simulink model "PVmodule"  (R2021a)
settings: Solver=VariableStepAuto  StartTime=0.0  StopTime=2.5  RelTol=1e-3
libraries: spsSeriesRLCBranchLib x2, pid_lib x2, spsMeanLib x2, spsDCVoltageSourceLib x1, spsDiodeLib x1, spsIGBTLib x1, eePwmGenerator x1, spsPVArrayLib x1, spsVoltageMeasurementLib x1, spspowerguiLib x1, SignalEditorBlockLib x1
settings Model: Creator=XieWHirlwind_TB  LastModifiedBy=XieWHirlwind_TB

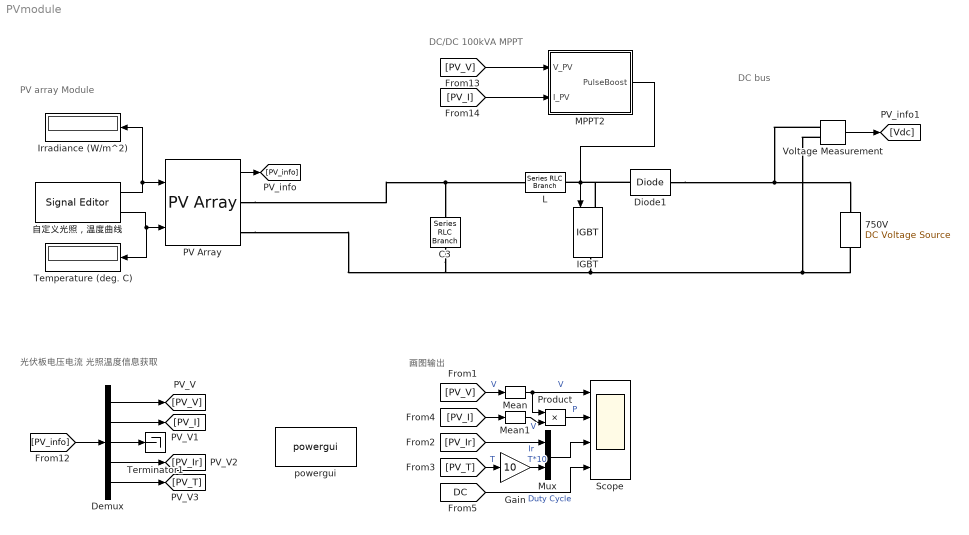
== system PVmodule ==
  note: DC bus
  note: 画图输出
  note: DC/DC 100kVA MPPT
  note: PV array Module
  note: 光伏板电压电流
      | 光照温度信息获取
  750V : spsDCVoltageSourceLib/DC Voltage Source  Amplitude=750  Measurements=None
  C3 : spsSeriesRLCBranchLib/Series RLC Branch  LConnTagsString=__new0  RConnTagsString=__new0  BranchType=C  Resistance=1.0  Inductance=1.0  SetiL0=off  InitialCurrent=0  Capacitance=470e-6  Setx0=off  InitialVoltage=0  Measurements=Branch voltage
  Demux : Demux  Outputs=5
  Diode1 : spsDiodeLib/Diode  Ron=1e-3  Lon=0  Vf=0.7  IC=0  UseSnubber=off  Rs=inf  Cs=inf  Measurements=off
  Gain : Gain  Gain=10
  IGBT : spsIGBTLib/IGBT  Ron=1e-3  Lon=0  Vf=0.7  Tf=1e-6  Tt=2e-6  IC=0  Rs=1e5  Cs=inf  Measurements=off
  Irradiance (W/m^2) : Display
      settings: Format=bank  Decimation=1000
  L : spsSeriesRLCBranchLib/Series RLC Branch  LConnTagsString=__new0  RConnTagsString=__new0  BranchType=RL  Resistance=0.0005  Inductance=1e-3  SetiL0=off  InitialCurrent=0  Capacitance=1e-6  Setx0=off  InitialVoltage=0  Measurements=None
  MPPT2 : Subsystem
  Mean : spsMeanLib/Mean  Freq=1e3  Vinit=0  Ts=1e-4
  Mean1 : spsMeanLib/Mean  Freq=1e3  Vinit=0  Ts=1e-4
  Mux : Mux  Inputs=2
  PV Array : spsPVArrayLib/PV Array  Npar=45  Nser=10  PlotType=array @ 25 deg.C & specified irradiances  S_vec="[ 1000 800 350  100 ]"  Temp_C_vec="[ 45 25  ]"  ModuleName=A2Peak Power POWER ON P220-6x10  PlotWhenSelected=off  Pm=219.978  Ncell=60  Voc=36.72  Isc=7.98  Vm=30.3  Im=7.26  beta_Voc_pc=-0.35  alpha_Isc_pc=0.05  beta_Voc=-0.12852  alpha_Isc=0.00399  IL=8.0041  I0=1.8441e-10  nI=0.97472  Rsh=85.0716  Rs=0.25728  RobustModel=off  RobustCellTemperature=313.3991  BAL=on  Tc=1e-6  Tfilter=5e-5
  Product : Product
  Scope : Scope  NumInputPorts=4
  Temperature (deg. C) : Display
      settings: Format=bank  Decimation=1000
  Terminator1 : Terminator
  Voltage Measurement : spsVoltageMeasurementLib/Voltage Measurement  PhasorSimulation=off  OutputType=Complex  PSBequivalent=0
  powergui : spspowerguiLib/powergui  Priority=1  SimulationMode=Discrete  SampleTime=2e-6  frequency=60  Iterations=50  frequencyindice=0  Pbase=100e6  ErrMax=1e-4  UnitsV=kV  UnitsW=MW  buscounter=0  FunctionMessages=off  echomessages=off  EnableUseOfTLC=off  CurrentSourceSwitches=off  DisableSnubberDevices=off  DisableRonSwitches=off  DisableVfSwitches=off  DisplayEquations=off  AutomaticDiscreteSolvers=off  SolverType=Tustin/Backward Euler (TBE)  Interpol=off  ExternalGateDelay=off  methode=off  Ts=100  x0status=blocks  SPID=on  SwTol=0  HookPort=off  NonlinearTolerance=1e-4  nMaxIteration=100  ContinueOnMaxIteration=off  RestoreLinks=warning  ResistiveCurrentMeasurement=off  Frange=[0:2:500]  Ylog=off  Xlog=on  ShowGrid=off  save=off  variable=ZData  structure=0  ZoomFFT=off  StartTime=0.0  cycles=1  DisplayStyle=1  fundamental=60  FreqAxis=off  MaxFrequency=1000  frequencyindicesteady=1  RmsSteady=1  display=off
  自定义光照，温度曲线 : SignalEditorBlockLib/Signal Editor  FileName=Irr_Temp_1.mat  ActiveScenario=Scenario1  ActiveSignal=Temp  IsBus=off  OutputBusObjectStr=Bus: BusObject  SampleTime=0  ZeroCross=off  OutputAfterFinalValue=Setting to zero  Unit=inherit  PreserveSignalName=on
  wires:
  MPPT2/1(PulseBoost) -> IGBT/1
  [PV_V] -> MPPT2/1(V_PV)
  自定义光照，温度曲线/2 -> Temperature (deg. C)/1, PV Array/2
  PV Array/1 -> [PV_info]
  自定义光照，温度曲线/1 -> Irradiance (W/m^2)/1, PV Array/1
  Demux/3 -> Terminator1/1
  Demux/4 -> [PV_Ir]
  Demux/5 -> [PV_T]
  [PV_info] -> Demux/1
  Demux/1 -> [PV_V]
  Demux/2 -> [PV_I]
  [PV_Ir] -> Mux/1  "Ir"
  Voltage Measurement/1 -> [Vdc]
  [PV_I] -> MPPT2/2(I_PV)
  Mean/1 -> Product/1, Scope/1  "V"
  [PV_V] -> Mean/1  "V"
  [PV_I] -> Mean1/1
  Product/1 -> Scope/2  "P"
  Mean1/1 -> Product/2  "V"
  Mux/1 -> Scope/3
  [DC] -> Scope/4  "Duty Cycle"
  [PV_T] -> Gain/1  "T"
  Gain/1 -> Mux/2  "T*10"
  connections:
  IGBT/RConn1 -- C3/RConn1 -- PV Array/RConn2 -- Voltage Measurement/LConn2 -- 750V/LConn1
  L/RConn1 -- IGBT/LConn1 -- Diode1/LConn1
  Diode1/RConn1 -- Voltage Measurement/LConn1 -- 750V/RConn1
  PV Array/RConn1 -- L/LConn1 -- C3/LConn1

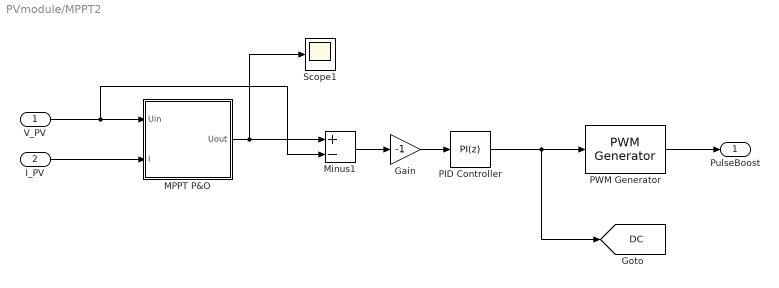
== system PVmodule/MPPT2 ==
  V_PV : Inport
  I_PV : Inport  Port=2
  Gain : Gain  Gain=-1
  MPPT P&O : Subsystem
  Minus1 : Sum  Inputs=+-
  PID Controller : pid_lib/PID Controller  Controller=PI  Form=Parallel  TimeDomain=Discrete-time  UseExternalTs=off  SampleTime=1e-4  IntegratorMethod=Forward Euler  FilterMethod=Forward Euler  ControllerParametersSource=internal  P=0.001  I=0.1  D=0  UseFilter=on  N=100  TunerSelectOption=Transfer Function Based (PID Tuner App)  InitialConditionSource=internal  InitialConditionForIntegrator=0  InitialConditionForFilter=0  DifferentiatorICPrevScaledInput=0  ExternalReset=none  TrackingMode=off  Kt=1  LimitOutput=on  SatLimitsSource=internal  UpperSaturationLimit=1  LowerSaturationLimit=0  LinearizeAsGain=on  AntiWindupMode=none  Kb=1  POutMin=[]  POutMax=[]  IOutMin=[]  IOutMax=[]  DOutMin=[]  DOutMax=[]  NOutMin=[]  NOutMax=[]  SumOutMin=[]  SumOutMax=[]  SaturationOutMin=[]  SaturationOutMax=[]  PParamMin=[]  PParamMax=[]  IParamMin=[]  IParamMax=[]  DParamMin=[]  DParamMax=[]  NParamMin=[]  NParamMax=[]  KbParamMin=[]  KbParamMax=[]  KtParamMin=[]  KtParamMax=[]  KbOutMin=[]  KbOutMax=[]  KtOutMin=[]  KtOutMax=[]  IntegratorOutMin=[]  IntegratorOutMax=[]  FilterOutMin=[]  FilterOutMax=[]  SumI1OutMin=[]  SumI1OutMax=[]  SumI2OutMin=[]  SumI2OutMax=[]  SumI3OutMin=[]  SumI3OutMax=[]  SumI4OutMin=[]  SumI4OutMax=[]  SumDOutMin=[]  SumDOutMax=[]  DifferentiatorOutMin=[]  DifferentiatorOutMax=[]  FilterDiffOutCoefMin=[]  FilterDiffOutCoefMax=[]  ReciprocalOutMin=[]  ReciprocalOutMax=[]  SumDenOutMin=[]  SumDenOutMax=[]  SumNumOutMin=[]  SumNumOutMax=[]  DivideOutMin=[]  DivideOutMax=[]  UdiffTsProdOutMin=[]  UdiffTsProdOutMax=[]  NTsProdOutMin=[]  NTsProdOutMax=[]  UintegralTsProdOutMin=[]  UintegralTsProdOutMax=[]  UngainTsProdOutMin=[]  UngainTsProdOutMax=[]  IntegratorContinuousStateAttributes=''  IntegratorStateMustResolveToSignalObject=off  IntegratorRTWStateStorageClass=Auto  FilterContinuousStateAttributes=''  FilterStateMustResolveToSignalObject=off  FilterRTWStateStorageClass=Auto  ParallelPVariant=InternalParameters  IdealPVariant=Disabled  IVariant=InternalParameters  DVariant=Disabled  IntegratorVariant=Discrete  SatVariant=Enabled  AWVariant=Passthrough  PCopyVariant=Disabled  TRVariant=Disabled  FdbkBlocksVariant=Forward  IdealPFdbkVariant=Disabled  SatFdbkVariant=Disabled  DerivativeFilterVariant=Disabled  NVariant=Disabled  NCopyVariant=Disabled_SignalSpec  FilterICVariant=Disabled  IntegratorICVariant=InternalICs  ExternalResetVariant=Disabled  TRSumVariant=Passthrough  SumFdbkVariant=Disabled  SumVariant=Sum_PI  TsampFilterVariant=InternalTs  TsampNgainVariant=Passthrough  TsampIntegralVariant=Passthrough  ExternalSaturationOutDataTypeStr=Inherit: Same as second input
  PWM Generator : eePwmGenerator/PWM Generator  CarrCount=Up  Tper=1e-4  Ts=2e-6
  Scope1 : Scope
  PulseBoost : Outport
  tag scope: DC=global
  wires:
  PWM Generator/1 -> PulseBoost/1
  I_PV/1 -> MPPT P&O/2(I)
  V_PV/1 -> Minus1/2, MPPT P&O/1(Uin)
  MPPT P&O/1(Uout) -> Minus1/1, Scope1/1
  Minus1/1 -> Gain/1
  PID Controller/1 -> [DC], PWM Generator/1
  Gain/1 -> PID Controller/1

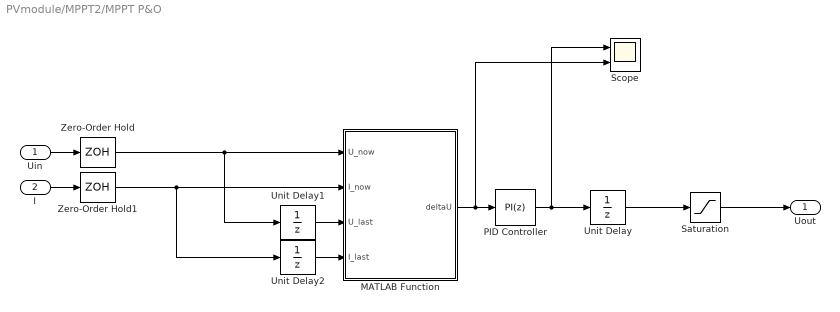
== system PVmodule/MPPT2/MPPT P&O ==
  Uin : Inport
  I : Inport  Port=2
  MATLAB Function : MATLAB Function  TreatAsAtomicUnit=on
  PID Controller : pid_lib/PID Controller  Controller=PI  Form=Parallel  TimeDomain=Discrete-time  UseExternalTs=off  SampleTime=1e-3  IntegratorMethod=Forward Euler  FilterMethod=Forward Euler  ControllerParametersSource=internal  P=1  I=100  D=0  UseFilter=on  N=100  TunerSelectOption=Transfer Function Based (PID Tuner App)  InitialConditionSource=internal  InitialConditionForIntegrator=250  InitialConditionForFilter=0  DifferentiatorICPrevScaledInput=0  ExternalReset=none  TrackingMode=off  Kt=1  LimitOutput=off  SatLimitsSource=internal  UpperSaturationLimit=inf  LowerSaturationLimit=-inf  LinearizeAsGain=on  AntiWindupMode=none  Kb=1  POutMin=[]  POutMax=[]  IOutMin=[]  IOutMax=[]  DOutMin=[]  DOutMax=[]  NOutMin=[]  NOutMax=[]  SumOutMin=[]  SumOutMax=[]  SaturationOutMin=[]  SaturationOutMax=[]  PParamMin=[]  PParamMax=[]  IParamMin=[]  IParamMax=[]  DParamMin=[]  DParamMax=[]  NParamMin=[]  NParamMax=[]  KbParamMin=[]  KbParamMax=[]  KtParamMin=[]  KtParamMax=[]  KbOutMin=[]  KbOutMax=[]  KtOutMin=[]  KtOutMax=[]  IntegratorOutMin=[]  IntegratorOutMax=[]  FilterOutMin=[]  FilterOutMax=[]  SumI1OutMin=[]  SumI1OutMax=[]  SumI2OutMin=[]  SumI2OutMax=[]  SumI3OutMin=[]  SumI3OutMax=[]  SumI4OutMin=[]  SumI4OutMax=[]  SumDOutMin=[]  SumDOutMax=[]  DifferentiatorOutMin=[]  DifferentiatorOutMax=[]  FilterDiffOutCoefMin=[]  FilterDiffOutCoefMax=[]  ReciprocalOutMin=[]  ReciprocalOutMax=[]  SumDenOutMin=[]  SumDenOutMax=[]  SumNumOutMin=[]  SumNumOutMax=[]  DivideOutMin=[]  DivideOutMax=[]  UdiffTsProdOutMin=[]  UdiffTsProdOutMax=[]  NTsProdOutMin=[]  NTsProdOutMax=[]  UintegralTsProdOutMin=[]  UintegralTsProdOutMax=[]  UngainTsProdOutMin=[]  UngainTsProdOutMax=[]  IntegratorContinuousStateAttributes=''  IntegratorStateMustResolveToSignalObject=off  IntegratorRTWStateStorageClass=Auto  FilterContinuousStateAttributes=''  FilterStateMustResolveToSignalObject=off  FilterRTWStateStorageClass=Auto  ParallelPVariant=InternalParameters  IdealPVariant=Disabled  IVariant=InternalParameters  DVariant=Disabled  IntegratorVariant=Discrete  SatVariant=Disabled  AWVariant=Passthrough  PCopyVariant=Disabled  TRVariant=Disabled  FdbkBlocksVariant=Forward  IdealPFdbkVariant=Disabled  SatFdbkVariant=Disabled  DerivativeFilterVariant=Disabled  NVariant=Disabled  NCopyVariant=Disabled_SignalSpec  FilterICVariant=Disabled  IntegratorICVariant=InternalICs  ExternalResetVariant=Disabled  TRSumVariant=Passthrough  SumFdbkVariant=Disabled  SumVariant=Sum_PI  TsampFilterVariant=InternalTs  TsampNgainVariant=Passthrough  TsampIntegralVariant=Passthrough  ExternalSaturationOutDataTypeStr=Inherit: Same as second input
  Saturation : Saturate  UpperLimit=360  LowerLimit=0
  Scope : Scope  NumInputPorts=2
  Unit Delay : UnitDelay  InitialCondition=250  SampleTime=1e-3  HasFrameUpgradeWarning=on
  Unit Delay1 : UnitDelay  InitialCondition=250  SampleTime=1e-3  HasFrameUpgradeWarning=on
  Unit Delay2 : UnitDelay  SampleTime=1e-3  HasFrameUpgradeWarning=on
  Zero-Order Hold : ZeroOrderHold  SampleTime=1e-3
  Zero-Order Hold1 : ZeroOrderHold  SampleTime=1e-3
  Uout : Outport
  wires:
  Unit Delay1/1 -> MATLAB Function/3(U_last)
  MATLAB Function/1(deltaU) -> PID Controller/1, Scope/2
  Unit Delay2/1 -> MATLAB Function/4(I_last)
  Unit Delay/1 -> Saturation/1
  Saturation/1 -> Uout/1
  I/1 -> Zero-Order Hold1/1
  Zero-Order Hold1/1 -> Unit Delay2/1, MATLAB Function/2(I_now)
  Uin/1 -> Zero-Order Hold/1
  Zero-Order Hold/1 -> Unit Delay1/1, MATLAB Function/1(U_now)
  PID Controller/1 -> Unit Delay/1, Scope/1

== matlab function PVmodule/MPPT2/MPPT P&O/MATLAB Function ==
  data: U_now input; deltaU output; I_now input; U_last input; I_last input
function deltaU  = MPPT_PandO(U_now, I_now, U_last, I_last)
    step = 5;
    %计算dP、dU
    dU = U_now - U_last;
    dP = U_now*I_now - U_last*I_last;
    
    if(dP == 0)
        deltaU = 0;
    else
        if(dP > 0)
            if(dU > 0)
                deltaU = 0 + step;
            else
                deltaU = 0 - step;
            end
        else
            if(dU > 0)
                deltaU = 0 - step;
            else
                deltaU = 0 + step;
            end
        end
    end
%     
%     if(dP == 0)
%         U_ref = U_now;
%     else
%         if(dP > 0)
%             if(dU > 0)
%                 U_ref = U_now + step;
%             else
%                 U_ref = U_now - step;
%             end
%         else
%             if(dU > 0)
%                 U_ref = U_now - step;
%             else
%                 U_ref = U_now + step;
%             end
%         end
%     end
